simulink model "gm_soc_dvbs2_fpga"  (R2025b)
settings: Solver=VariableStepAuto  StartTime=0.0  StopTime=10.0  RelTol=1e-3
InitFcn:
  | soc_dvbs2_init;
undefined symbols (not defined in the file or in its folder): Add, coefficientsLog, coefficientsSqrt1, coefficientsSqrt2, dataBits, Deinterleaver, designMultirateFIR, noisePow, Shift, Short, soc_dvbs2_designFIRFilter, soc_dvbs2_txPacketBits, syncWord, txDataOut, txFiltCoeff, XData
libraries: simulink x304, hdlsllib x265, dspsigops x15, dsphdlfiltering2 x8, hdlmdlgenlib x6, dsphdlsigops2 x5, commseqgen3 x5, dsphdlmathfun2 x3, hwlogicconnlib x2, whdledac x2, commhdlcrc x2, whdlutilities x1
(part 27 of 36)

== system gm_soc_dvbs2_fpga/DVBS2/DVBS2 TxRx/DVB-S2 HDL Receiver/Synchronizer and PL Header Decoder/PL Header Recovery/PL Header Decoder/ML Decoder/Euclidean Distance Sum Up_instance55 ==
  note: For Each
  Ed0 : Inport  OutDataTypeStr=fixdt(1, 25, 15)  PortDimensions=1  SampleTime=2.5e-07
  Ed1 : Inport  Port=2  OutDataTypeStr=fixdt(1, 20, 13)  PortDimensions=1  SampleTime=2.5e-07
  reset : Inport  Port=3  OutDataTypeStr=boolean  PortDimensions=1  SampleTime=2.5e-07
  CWswitch : Inport  Port=4  OutDataTypeStr=fixdt(0, 1, 0)  PortDimensions=1  SampleTime=2.5e-07
  validIn : Inport  Port=5  OutDataTypeStr=boolean  PortDimensions=1  SampleTime=2.5e-07
  Add : Sum  OutDataTypeStr=fixdt(1, 25, 15)  AccumDataTypeStr=fixdt(1, 26, 15)  SampleTime=2.5e-07
  Delay{1..4} (4 alike) : Delay  DelayLength=double(1)  InitialCondition=0  SampleTime=2.5e-07
  Switch : Switch  Criteria=u2 ~= 0  Threshold="fi(0,0,1,0,\"hex\",\"0\")"  OutDataTypeStr=fixdt(1, 25, 15)  SampleTime=2.5e-07  SaturateOnIntegerOverflow=off  InputSameDT=off
  Unit Delay Enabled Resettable Synchronous : hdlsllib/Discrete/Unit Delay Enabled Resettable Synchronous  InitialCondition=double(0)  SampleTime=-1
  CwEdMetric : Outport  SampleTime=2.5e-07
  wires:
  Switch/1 -> Delay3/1
  validIn/1 -> Delay1/1
  Delay1/1 -> Unit Delay Enabled Resettable Synchronous/2
  Ed0/1 -> Switch/3
  reset/1 -> Delay2/1
  CWswitch/1 -> Switch/2
  Ed1/1 -> Switch/1
  Delay2/1 -> Unit Delay Enabled Resettable Synchronous/3
  Unit Delay Enabled Resettable Synchronous/1 -> Delay4/1, Add/1
  Add/1 -> Unit Delay Enabled Resettable Synchronous/1
  Delay3/1 -> Add/2
  Delay4/1 -> CwEdMetric/1

== system gm_soc_dvbs2_fpga/DVBS2/DVBS2 TxRx/DVB-S2 HDL Receiver/Synchronizer and PL Header Decoder/PL Header Recovery/PL Header Decoder/ML Decoder/Euclidean Distance Sum Up_instance56 ==
  note: For Each
  Ed0 : Inport  OutDataTypeStr=fixdt(1, 25, 15)  PortDimensions=1  SampleTime=2.5e-07
  Ed1 : Inport  Port=2  OutDataTypeStr=fixdt(1, 20, 13)  PortDimensions=1  SampleTime=2.5e-07
  reset : Inport  Port=3  OutDataTypeStr=boolean  PortDimensions=1  SampleTime=2.5e-07
  CWswitch : Inport  Port=4  OutDataTypeStr=fixdt(0, 1, 0)  PortDimensions=1  SampleTime=2.5e-07
  validIn : Inport  Port=5  OutDataTypeStr=boolean  PortDimensions=1  SampleTime=2.5e-07
  Add : Sum  OutDataTypeStr=fixdt(1, 25, 15)  AccumDataTypeStr=fixdt(1, 26, 15)  SampleTime=2.5e-07
  Delay{1..4} (4 alike) : Delay  DelayLength=double(1)  InitialCondition=0  SampleTime=2.5e-07
  Switch : Switch  Criteria=u2 ~= 0  Threshold="fi(0,0,1,0,\"hex\",\"0\")"  OutDataTypeStr=fixdt(1, 25, 15)  SampleTime=2.5e-07  SaturateOnIntegerOverflow=off  InputSameDT=off
  Unit Delay Enabled Resettable Synchronous : hdlsllib/Discrete/Unit Delay Enabled Resettable Synchronous  InitialCondition=double(0)  SampleTime=-1
  CwEdMetric : Outport  SampleTime=2.5e-07
  wires:
  validIn/1 -> Delay1/1
  Delay1/1 -> Unit Delay Enabled Resettable Synchronous/2
  Ed0/1 -> Switch/3
  reset/1 -> Delay2/1
  Delay2/1 -> Unit Delay Enabled Resettable Synchronous/3
  CWswitch/1 -> Switch/2
  Ed1/1 -> Switch/1
  Switch/1 -> Delay3/1
  Unit Delay Enabled Resettable Synchronous/1 -> Delay4/1, Add/1
  Delay3/1 -> Add/2
  Delay4/1 -> CwEdMetric/1
  Add/1 -> Unit Delay Enabled Resettable Synchronous/1

== system gm_soc_dvbs2_fpga/DVBS2/DVBS2 TxRx/DVB-S2 HDL Receiver/Synchronizer and PL Header Decoder/PL Header Recovery/PL Header Decoder/ML Decoder/Euclidean Distance Sum Up_instance57 ==
  note: For Each
  Ed0 : Inport  OutDataTypeStr=fixdt(1, 25, 15)  PortDimensions=1  SampleTime=2.5e-07
  Ed1 : Inport  Port=2  OutDataTypeStr=fixdt(1, 20, 13)  PortDimensions=1  SampleTime=2.5e-07
  reset : Inport  Port=3  OutDataTypeStr=boolean  PortDimensions=1  SampleTime=2.5e-07
  CWswitch : Inport  Port=4  OutDataTypeStr=fixdt(0, 1, 0)  PortDimensions=1  SampleTime=2.5e-07
  validIn : Inport  Port=5  OutDataTypeStr=boolean  PortDimensions=1  SampleTime=2.5e-07
  Add : Sum  OutDataTypeStr=fixdt(1, 25, 15)  AccumDataTypeStr=fixdt(1, 26, 15)  SampleTime=2.5e-07
  Delay{1..4} (4 alike) : Delay  DelayLength=double(1)  InitialCondition=0  SampleTime=2.5e-07
  Switch : Switch  Criteria=u2 ~= 0  Threshold="fi(0,0,1,0,\"hex\",\"0\")"  OutDataTypeStr=fixdt(1, 25, 15)  SampleTime=2.5e-07  SaturateOnIntegerOverflow=off  InputSameDT=off
  Unit Delay Enabled Resettable Synchronous : hdlsllib/Discrete/Unit Delay Enabled Resettable Synchronous  InitialCondition=double(0)  SampleTime=-1
  CwEdMetric : Outport  SampleTime=2.5e-07
  wires:
  Switch/1 -> Delay3/1
  validIn/1 -> Delay1/1
  Delay1/1 -> Unit Delay Enabled Resettable Synchronous/2
  Ed0/1 -> Switch/3
  reset/1 -> Delay2/1
  CWswitch/1 -> Switch/2
  Ed1/1 -> Switch/1
  Delay2/1 -> Unit Delay Enabled Resettable Synchronous/3
  Unit Delay Enabled Resettable Synchronous/1 -> Delay4/1, Add/1
  Add/1 -> Unit Delay Enabled Resettable Synchronous/1
  Delay3/1 -> Add/2
  Delay4/1 -> CwEdMetric/1

== system gm_soc_dvbs2_fpga/DVBS2/DVBS2 TxRx/DVB-S2 HDL Receiver/Synchronizer and PL Header Decoder/PL Header Recovery/PL Header Decoder/ML Decoder/Euclidean Distance Sum Up_instance58 ==
  note: For Each
  Ed0 : Inport  OutDataTypeStr=fixdt(1, 25, 15)  PortDimensions=1  SampleTime=2.5e-07
  Ed1 : Inport  Port=2  OutDataTypeStr=fixdt(1, 20, 13)  PortDimensions=1  SampleTime=2.5e-07
  reset : Inport  Port=3  OutDataTypeStr=boolean  PortDimensions=1  SampleTime=2.5e-07
  CWswitch : Inport  Port=4  OutDataTypeStr=fixdt(0, 1, 0)  PortDimensions=1  SampleTime=2.5e-07
  validIn : Inport  Port=5  OutDataTypeStr=boolean  PortDimensions=1  SampleTime=2.5e-07
  Add : Sum  OutDataTypeStr=fixdt(1, 25, 15)  AccumDataTypeStr=fixdt(1, 26, 15)  SampleTime=2.5e-07
  Delay{1..4} (4 alike) : Delay  DelayLength=double(1)  InitialCondition=0  SampleTime=2.5e-07
  Switch : Switch  Criteria=u2 ~= 0  Threshold="fi(0,0,1,0,\"hex\",\"0\")"  OutDataTypeStr=fixdt(1, 25, 15)  SampleTime=2.5e-07  SaturateOnIntegerOverflow=off  InputSameDT=off
  Unit Delay Enabled Resettable Synchronous : hdlsllib/Discrete/Unit Delay Enabled Resettable Synchronous  InitialCondition=double(0)  SampleTime=-1
  CwEdMetric : Outport  SampleTime=2.5e-07
  wires:
  Switch/1 -> Delay3/1
  validIn/1 -> Delay1/1
  Delay1/1 -> Unit Delay Enabled Resettable Synchronous/2
  Ed0/1 -> Switch/3
  reset/1 -> Delay2/1
  Delay2/1 -> Unit Delay Enabled Resettable Synchronous/3
  CWswitch/1 -> Switch/2
  Ed1/1 -> Switch/1
  Unit Delay Enabled Resettable Synchronous/1 -> Delay4/1, Add/1
  Delay3/1 -> Add/2
  Delay4/1 -> CwEdMetric/1
  Add/1 -> Unit Delay Enabled Resettable Synchronous/1

== system gm_soc_dvbs2_fpga/DVBS2/DVBS2 TxRx/DVB-S2 HDL Receiver/Synchronizer and PL Header Decoder/PL Header Recovery/PL Header Decoder/ML Decoder/Euclidean Distance Sum Up_instance59 ==
  note: For Each
  Ed0 : Inport  OutDataTypeStr=fixdt(1, 25, 15)  PortDimensions=1  SampleTime=2.5e-07
  Ed1 : Inport  Port=2  OutDataTypeStr=fixdt(1, 20, 13)  PortDimensions=1  SampleTime=2.5e-07
  reset : Inport  Port=3  OutDataTypeStr=boolean  PortDimensions=1  SampleTime=2.5e-07
  CWswitch : Inport  Port=4  OutDataTypeStr=fixdt(0, 1, 0)  PortDimensions=1  SampleTime=2.5e-07
  validIn : Inport  Port=5  OutDataTypeStr=boolean  PortDimensions=1  SampleTime=2.5e-07
  Add : Sum  OutDataTypeStr=fixdt(1, 25, 15)  AccumDataTypeStr=fixdt(1, 26, 15)  SampleTime=2.5e-07
  Delay{1..4} (4 alike) : Delay  DelayLength=double(1)  InitialCondition=0  SampleTime=2.5e-07
  Switch : Switch  Criteria=u2 ~= 0  Threshold="fi(0,0,1,0,\"hex\",\"0\")"  OutDataTypeStr=fixdt(1, 25, 15)  SampleTime=2.5e-07  SaturateOnIntegerOverflow=off  InputSameDT=off
  Unit Delay Enabled Resettable Synchronous : hdlsllib/Discrete/Unit Delay Enabled Resettable Synchronous  InitialCondition=double(0)  SampleTime=-1
  CwEdMetric : Outport  SampleTime=2.5e-07
  wires:
  Switch/1 -> Delay3/1
  validIn/1 -> Delay1/1
  Delay1/1 -> Unit Delay Enabled Resettable Synchronous/2
  Ed0/1 -> Switch/3
  reset/1 -> Delay2/1
  CWswitch/1 -> Switch/2
  Ed1/1 -> Switch/1
  Delay2/1 -> Unit Delay Enabled Resettable Synchronous/3
  Unit Delay Enabled Resettable Synchronous/1 -> Add/1, Delay4/1
  Add/1 -> Unit Delay Enabled Resettable Synchronous/1
  Delay3/1 -> Add/2
  Delay4/1 -> CwEdMetric/1

== system gm_soc_dvbs2_fpga/DVBS2/DVBS2 TxRx/DVB-S2 HDL Receiver/Synchronizer and PL Header Decoder/PL Header Recovery/PL Header Decoder/ML Decoder/Euclidean Distance Sum Up_instance6 ==
  note: For Each
  Ed0 : Inport  OutDataTypeStr=fixdt(1, 25, 15)  PortDimensions=1  SampleTime=2.5e-07
  Ed1 : Inport  Port=2  OutDataTypeStr=fixdt(1, 20, 13)  PortDimensions=1  SampleTime=2.5e-07
  reset : Inport  Port=3  OutDataTypeStr=boolean  PortDimensions=1  SampleTime=2.5e-07
  CWswitch : Inport  Port=4  OutDataTypeStr=fixdt(0, 1, 0)  PortDimensions=1  SampleTime=2.5e-07
  validIn : Inport  Port=5  OutDataTypeStr=boolean  PortDimensions=1  SampleTime=2.5e-07
  Add : Sum  OutDataTypeStr=fixdt(1, 25, 15)  AccumDataTypeStr=fixdt(1, 26, 15)  SampleTime=2.5e-07
  Delay{1..4} (4 alike) : Delay  DelayLength=double(1)  InitialCondition=0  SampleTime=2.5e-07
  Switch : Switch  Criteria=u2 ~= 0  Threshold="fi(0,0,1,0,\"hex\",\"0\")"  OutDataTypeStr=fixdt(1, 25, 15)  SampleTime=2.5e-07  SaturateOnIntegerOverflow=off  InputSameDT=off
  Unit Delay Enabled Resettable Synchronous : hdlsllib/Discrete/Unit Delay Enabled Resettable Synchronous  InitialCondition=double(0)  SampleTime=-1
  CwEdMetric : Outport  SampleTime=2.5e-07
  wires:
  Switch/1 -> Delay3/1
  validIn/1 -> Delay1/1
  Delay1/1 -> Unit Delay Enabled Resettable Synchronous/2
  Ed0/1 -> Switch/3
  reset/1 -> Delay2/1
  Delay2/1 -> Unit Delay Enabled Resettable Synchronous/3
  CWswitch/1 -> Switch/2
  Ed1/1 -> Switch/1
  Unit Delay Enabled Resettable Synchronous/1 -> Delay4/1, Add/1
  Add/1 -> Unit Delay Enabled Resettable Synchronous/1
  Delay3/1 -> Add/2
  Delay4/1 -> CwEdMetric/1

== system gm_soc_dvbs2_fpga/DVBS2/DVBS2 TxRx/DVB-S2 HDL Receiver/Synchronizer and PL Header Decoder/PL Header Recovery/PL Header Decoder/ML Decoder/Euclidean Distance Sum Up_instance60 ==
  note: For Each
  Ed0 : Inport  OutDataTypeStr=fixdt(1, 25, 15)  PortDimensions=1  SampleTime=2.5e-07
  Ed1 : Inport  Port=2  OutDataTypeStr=fixdt(1, 20, 13)  PortDimensions=1  SampleTime=2.5e-07
  reset : Inport  Port=3  OutDataTypeStr=boolean  PortDimensions=1  SampleTime=2.5e-07
  CWswitch : Inport  Port=4  OutDataTypeStr=fixdt(0, 1, 0)  PortDimensions=1  SampleTime=2.5e-07
  validIn : Inport  Port=5  OutDataTypeStr=boolean  PortDimensions=1  SampleTime=2.5e-07
  Add : Sum  OutDataTypeStr=fixdt(1, 25, 15)  AccumDataTypeStr=fixdt(1, 26, 15)  SampleTime=2.5e-07
  Delay{1..4} (4 alike) : Delay  DelayLength=double(1)  InitialCondition=0  SampleTime=2.5e-07
  Switch : Switch  Criteria=u2 ~= 0  Threshold="fi(0,0,1,0,\"hex\",\"0\")"  OutDataTypeStr=fixdt(1, 25, 15)  SampleTime=2.5e-07  SaturateOnIntegerOverflow=off  InputSameDT=off
  Unit Delay Enabled Resettable Synchronous : hdlsllib/Discrete/Unit Delay Enabled Resettable Synchronous  InitialCondition=double(0)  SampleTime=-1
  CwEdMetric : Outport  SampleTime=2.5e-07
  wires:
  Switch/1 -> Delay3/1
  validIn/1 -> Delay1/1
  Delay1/1 -> Unit Delay Enabled Resettable Synchronous/2
  Ed0/1 -> Switch/3
  reset/1 -> Delay2/1
  Delay2/1 -> Unit Delay Enabled Resettable Synchronous/3
  CWswitch/1 -> Switch/2
  Ed1/1 -> Switch/1
  Unit Delay Enabled Resettable Synchronous/1 -> Delay4/1, Add/1
  Delay3/1 -> Add/2
  Delay4/1 -> CwEdMetric/1
  Add/1 -> Unit Delay Enabled Resettable Synchronous/1

== system gm_soc_dvbs2_fpga/DVBS2/DVBS2 TxRx/DVB-S2 HDL Receiver/Synchronizer and PL Header Decoder/PL Header Recovery/PL Header Decoder/ML Decoder/Euclidean Distance Sum Up_instance61 ==
  note: For Each
  Ed0 : Inport  OutDataTypeStr=fixdt(1, 25, 15)  PortDimensions=1  SampleTime=2.5e-07
  Ed1 : Inport  Port=2  OutDataTypeStr=fixdt(1, 20, 13)  PortDimensions=1  SampleTime=2.5e-07
  reset : Inport  Port=3  OutDataTypeStr=boolean  PortDimensions=1  SampleTime=2.5e-07
  CWswitch : Inport  Port=4  OutDataTypeStr=fixdt(0, 1, 0)  PortDimensions=1  SampleTime=2.5e-07
  validIn : Inport  Port=5  OutDataTypeStr=boolean  PortDimensions=1  SampleTime=2.5e-07
  Add : Sum  OutDataTypeStr=fixdt(1, 25, 15)  AccumDataTypeStr=fixdt(1, 26, 15)  SampleTime=2.5e-07
  Delay{1..4} (4 alike) : Delay  DelayLength=double(1)  InitialCondition=0  SampleTime=2.5e-07
  Switch : Switch  Criteria=u2 ~= 0  Threshold="fi(0,0,1,0,\"hex\",\"0\")"  OutDataTypeStr=fixdt(1, 25, 15)  SampleTime=2.5e-07  SaturateOnIntegerOverflow=off  InputSameDT=off
  Unit Delay Enabled Resettable Synchronous : hdlsllib/Discrete/Unit Delay Enabled Resettable Synchronous  InitialCondition=double(0)  SampleTime=-1
  CwEdMetric : Outport  SampleTime=2.5e-07
  wires:
  Switch/1 -> Delay3/1
  validIn/1 -> Delay1/1
  Delay1/1 -> Unit Delay Enabled Resettable Synchronous/2
  Ed0/1 -> Switch/3
  reset/1 -> Delay2/1
  CWswitch/1 -> Switch/2
  Ed1/1 -> Switch/1
  Delay2/1 -> Unit Delay Enabled Resettable Synchronous/3
  Unit Delay Enabled Resettable Synchronous/1 -> Delay4/1, Add/1
  Add/1 -> Unit Delay Enabled Resettable Synchronous/1
  Delay3/1 -> Add/2
  Delay4/1 -> CwEdMetric/1

== system gm_soc_dvbs2_fpga/DVBS2/DVBS2 TxRx/DVB-S2 HDL Receiver/Synchronizer and PL Header Decoder/PL Header Recovery/PL Header Decoder/ML Decoder/Euclidean Distance Sum Up_instance62 ==
  note: For Each
  Ed0 : Inport  OutDataTypeStr=fixdt(1, 25, 15)  PortDimensions=1  SampleTime=2.5e-07
  Ed1 : Inport  Port=2  OutDataTypeStr=fixdt(1, 20, 13)  PortDimensions=1  SampleTime=2.5e-07
  reset : Inport  Port=3  OutDataTypeStr=boolean  PortDimensions=1  SampleTime=2.5e-07
  CWswitch : Inport  Port=4  OutDataTypeStr=fixdt(0, 1, 0)  PortDimensions=1  SampleTime=2.5e-07
  validIn : Inport  Port=5  OutDataTypeStr=boolean  PortDimensions=1  SampleTime=2.5e-07
  Add : Sum  OutDataTypeStr=fixdt(1, 25, 15)  AccumDataTypeStr=fixdt(1, 26, 15)  SampleTime=2.5e-07
  Delay{1..4} (4 alike) : Delay  DelayLength=double(1)  InitialCondition=0  SampleTime=2.5e-07
  Switch : Switch  Criteria=u2 ~= 0  Threshold="fi(0,0,1,0,\"hex\",\"0\")"  OutDataTypeStr=fixdt(1, 25, 15)  SampleTime=2.5e-07  SaturateOnIntegerOverflow=off  InputSameDT=off
  Unit Delay Enabled Resettable Synchronous : hdlsllib/Discrete/Unit Delay Enabled Resettable Synchronous  InitialCondition=double(0)  SampleTime=-1
  CwEdMetric : Outport  SampleTime=2.5e-07
  wires:
  Switch/1 -> Delay3/1
  validIn/1 -> Delay1/1
  Delay1/1 -> Unit Delay Enabled Resettable Synchronous/2
  Ed0/1 -> Switch/3
  reset/1 -> Delay2/1
  Delay2/1 -> Unit Delay Enabled Resettable Synchronous/3
  CWswitch/1 -> Switch/2
  Ed1/1 -> Switch/1
  Unit Delay Enabled Resettable Synchronous/1 -> Add/1, Delay4/1
  Add/1 -> Unit Delay Enabled Resettable Synchronous/1
  Delay3/1 -> Add/2
  Delay4/1 -> CwEdMetric/1

== system gm_soc_dvbs2_fpga/DVBS2/DVBS2 TxRx/DVB-S2 HDL Receiver/Synchronizer and PL Header Decoder/PL Header Recovery/PL Header Decoder/ML Decoder/Euclidean Distance Sum Up_instance63 ==
  note: For Each
  Ed0 : Inport  OutDataTypeStr=fixdt(1, 25, 15)  PortDimensions=1  SampleTime=2.5e-07
  Ed1 : Inport  Port=2  OutDataTypeStr=fixdt(1, 20, 13)  PortDimensions=1  SampleTime=2.5e-07
  reset : Inport  Port=3  OutDataTypeStr=boolean  PortDimensions=1  SampleTime=2.5e-07
  CWswitch : Inport  Port=4  OutDataTypeStr=fixdt(0, 1, 0)  PortDimensions=1  SampleTime=2.5e-07
  validIn : Inport  Port=5  OutDataTypeStr=boolean  PortDimensions=1  SampleTime=2.5e-07
  Add : Sum  OutDataTypeStr=fixdt(1, 25, 15)  AccumDataTypeStr=fixdt(1, 26, 15)  SampleTime=2.5e-07
  Delay{1..4} (4 alike) : Delay  DelayLength=double(1)  InitialCondition=0  SampleTime=2.5e-07
  Switch : Switch  Criteria=u2 ~= 0  Threshold="fi(0,0,1,0,\"hex\",\"0\")"  OutDataTypeStr=fixdt(1, 25, 15)  SampleTime=2.5e-07  SaturateOnIntegerOverflow=off  InputSameDT=off
  Unit Delay Enabled Resettable Synchronous : hdlsllib/Discrete/Unit Delay Enabled Resettable Synchronous  InitialCondition=double(0)  SampleTime=-1
  CwEdMetric : Outport  SampleTime=2.5e-07
  wires:
  Switch/1 -> Delay3/1
  validIn/1 -> Delay1/1
  Delay1/1 -> Unit Delay Enabled Resettable Synchronous/2
  Ed0/1 -> Switch/3
  reset/1 -> Delay2/1
  CWswitch/1 -> Switch/2
  Ed1/1 -> Switch/1
  Delay2/1 -> Unit Delay Enabled Resettable Synchronous/3
  Unit Delay Enabled Resettable Synchronous/1 -> Add/1, Delay4/1
  Add/1 -> Unit Delay Enabled Resettable Synchronous/1
  Delay3/1 -> Add/2
  Delay4/1 -> CwEdMetric/1

== system gm_soc_dvbs2_fpga/DVBS2/DVBS2 TxRx/DVB-S2 HDL Receiver/Synchronizer and PL Header Decoder/PL Header Recovery/PL Header Decoder/ML Decoder/Euclidean Distance Sum Up_instance64 ==
  note: For Each
  Ed0 : Inport  OutDataTypeStr=fixdt(1, 25, 15)  PortDimensions=1  SampleTime=2.5e-07
  Ed1 : Inport  Port=2  OutDataTypeStr=fixdt(1, 20, 13)  PortDimensions=1  SampleTime=2.5e-07
  reset : Inport  Port=3  OutDataTypeStr=boolean  PortDimensions=1  SampleTime=2.5e-07
  CWswitch : Inport  Port=4  OutDataTypeStr=fixdt(0, 1, 0)  PortDimensions=1  SampleTime=2.5e-07
  validIn : Inport  Port=5  OutDataTypeStr=boolean  PortDimensions=1  SampleTime=2.5e-07
  Add : Sum  OutDataTypeStr=fixdt(1, 25, 15)  AccumDataTypeStr=fixdt(1, 26, 15)  SampleTime=2.5e-07
  Delay{1..4} (4 alike) : Delay  DelayLength=double(1)  InitialCondition=0  SampleTime=2.5e-07
  Switch : Switch  Criteria=u2 ~= 0  Threshold="fi(0,0,1,0,\"hex\",\"0\")"  OutDataTypeStr=fixdt(1, 25, 15)  SampleTime=2.5e-07  SaturateOnIntegerOverflow=off  InputSameDT=off
  Unit Delay Enabled Resettable Synchronous : hdlsllib/Discrete/Unit Delay Enabled Resettable Synchronous  InitialCondition=double(0)  SampleTime=-1
  CwEdMetric : Outport  SampleTime=2.5e-07
  wires:
  Switch/1 -> Delay3/1
  validIn/1 -> Delay1/1
  Delay1/1 -> Unit Delay Enabled Resettable Synchronous/2
  Ed0/1 -> Switch/3
  reset/1 -> Delay2/1
  Delay2/1 -> Unit Delay Enabled Resettable Synchronous/3
  CWswitch/1 -> Switch/2
  Ed1/1 -> Switch/1
  Unit Delay Enabled Resettable Synchronous/1 -> Delay4/1, Add/1
  Add/1 -> Unit Delay Enabled Resettable Synchronous/1
  Delay3/1 -> Add/2
  Delay4/1 -> CwEdMetric/1

== system gm_soc_dvbs2_fpga/DVBS2/DVBS2 TxRx/DVB-S2 HDL Receiver/Synchronizer and PL Header Decoder/PL Header Recovery/PL Header Decoder/ML Decoder/Euclidean Distance Sum Up_instance7 ==
  note: For Each
  Ed0 : Inport  OutDataTypeStr=fixdt(1, 25, 15)  PortDimensions=1  SampleTime=2.5e-07
  Ed1 : Inport  Port=2  OutDataTypeStr=fixdt(1, 20, 13)  PortDimensions=1  SampleTime=2.5e-07
  reset : Inport  Port=3  OutDataTypeStr=boolean  PortDimensions=1  SampleTime=2.5e-07
  CWswitch : Inport  Port=4  OutDataTypeStr=fixdt(0, 1, 0)  PortDimensions=1  SampleTime=2.5e-07
  validIn : Inport  Port=5  OutDataTypeStr=boolean  PortDimensions=1  SampleTime=2.5e-07
  Add : Sum  OutDataTypeStr=fixdt(1, 25, 15)  AccumDataTypeStr=fixdt(1, 26, 15)  SampleTime=2.5e-07
  Delay{1..4} (4 alike) : Delay  DelayLength=double(1)  InitialCondition=0  SampleTime=2.5e-07
  Switch : Switch  Criteria=u2 ~= 0  Threshold="fi(0,0,1,0,\"hex\",\"0\")"  OutDataTypeStr=fixdt(1, 25, 15)  SampleTime=2.5e-07  SaturateOnIntegerOverflow=off  InputSameDT=off
  Unit Delay Enabled Resettable Synchronous : hdlsllib/Discrete/Unit Delay Enabled Resettable Synchronous  InitialCondition=double(0)  SampleTime=-1
  CwEdMetric : Outport  SampleTime=2.5e-07
  wires:
  Ed0/1 -> Switch/3
  reset/1 -> Delay2/1
  validIn/1 -> Delay1/1
  CWswitch/1 -> Switch/2
  Ed1/1 -> Switch/1
  Switch/1 -> Delay3/1
  Delay1/1 -> Unit Delay Enabled Resettable Synchronous/2
  Delay2/1 -> Unit Delay Enabled Resettable Synchronous/3
  Unit Delay Enabled Resettable Synchronous/1 -> Delay4/1, Add/1
  Add/1 -> Unit Delay Enabled Resettable Synchronous/1
  Delay3/1 -> Add/2
  Delay4/1 -> CwEdMetric/1

== system gm_soc_dvbs2_fpga/DVBS2/DVBS2 TxRx/DVB-S2 HDL Receiver/Synchronizer and PL Header Decoder/PL Header Recovery/PL Header Decoder/ML Decoder/Euclidean Distance Sum Up_instance8 ==
  note: For Each
  Ed0 : Inport  OutDataTypeStr=fixdt(1, 25, 15)  PortDimensions=1  SampleTime=2.5e-07
  Ed1 : Inport  Port=2  OutDataTypeStr=fixdt(1, 20, 13)  PortDimensions=1  SampleTime=2.5e-07
  reset : Inport  Port=3  OutDataTypeStr=boolean  PortDimensions=1  SampleTime=2.5e-07
  CWswitch : Inport  Port=4  OutDataTypeStr=fixdt(0, 1, 0)  PortDimensions=1  SampleTime=2.5e-07
  validIn : Inport  Port=5  OutDataTypeStr=boolean  PortDimensions=1  SampleTime=2.5e-07
  Add : Sum  OutDataTypeStr=fixdt(1, 25, 15)  AccumDataTypeStr=fixdt(1, 26, 15)  SampleTime=2.5e-07
  Delay{1..4} (4 alike) : Delay  DelayLength=double(1)  InitialCondition=0  SampleTime=2.5e-07
  Switch : Switch  Criteria=u2 ~= 0  Threshold="fi(0,0,1,0,\"hex\",\"0\")"  OutDataTypeStr=fixdt(1, 25, 15)  SampleTime=2.5e-07  SaturateOnIntegerOverflow=off  InputSameDT=off
  Unit Delay Enabled Resettable Synchronous : hdlsllib/Discrete/Unit Delay Enabled Resettable Synchronous  InitialCondition=double(0)  SampleTime=-1
  CwEdMetric : Outport  SampleTime=2.5e-07
  wires:
  Switch/1 -> Delay3/1
  validIn/1 -> Delay1/1
  Delay1/1 -> Unit Delay Enabled Resettable Synchronous/2
  Ed0/1 -> Switch/3
  reset/1 -> Delay2/1
  Delay2/1 -> Unit Delay Enabled Resettable Synchronous/3
  CWswitch/1 -> Switch/2
  Ed1/1 -> Switch/1
  Unit Delay Enabled Resettable Synchronous/1 -> Delay4/1, Add/1
  Add/1 -> Unit Delay Enabled Resettable Synchronous/1
  Delay3/1 -> Add/2
  Delay4/1 -> CwEdMetric/1

== system gm_soc_dvbs2_fpga/DVBS2/DVBS2 TxRx/DVB-S2 HDL Receiver/Synchronizer and PL Header Decoder/PL Header Recovery/PL Header Decoder/ML Decoder/Euclidean Distance Sum Up_instance9 ==
  note: For Each
  Ed0 : Inport  OutDataTypeStr=fixdt(1, 25, 15)  PortDimensions=1  SampleTime=2.5e-07
  Ed1 : Inport  Port=2  OutDataTypeStr=fixdt(1, 20, 13)  PortDimensions=1  SampleTime=2.5e-07
  reset : Inport  Port=3  OutDataTypeStr=boolean  PortDimensions=1  SampleTime=2.5e-07
  CWswitch : Inport  Port=4  OutDataTypeStr=fixdt(0, 1, 0)  PortDimensions=1  SampleTime=2.5e-07
  validIn : Inport  Port=5  OutDataTypeStr=boolean  PortDimensions=1  SampleTime=2.5e-07
  Add : Sum  OutDataTypeStr=fixdt(1, 25, 15)  AccumDataTypeStr=fixdt(1, 26, 15)  SampleTime=2.5e-07
  Delay{1..4} (4 alike) : Delay  DelayLength=double(1)  InitialCondition=0  SampleTime=2.5e-07
  Switch : Switch  Criteria=u2 ~= 0  Threshold="fi(0,0,1,0,\"hex\",\"0\")"  OutDataTypeStr=fixdt(1, 25, 15)  SampleTime=2.5e-07  SaturateOnIntegerOverflow=off  InputSameDT=off
  Unit Delay Enabled Resettable Synchronous : hdlsllib/Discrete/Unit Delay Enabled Resettable Synchronous  InitialCondition=double(0)  SampleTime=-1
  CwEdMetric : Outport  SampleTime=2.5e-07
  wires:
  Ed0/1 -> Switch/3
  reset/1 -> Delay2/1
  validIn/1 -> Delay1/1
  CWswitch/1 -> Switch/2
  Ed1/1 -> Switch/1
  Switch/1 -> Delay3/1
  Delay1/1 -> Unit Delay Enabled Resettable Synchronous/2
  Delay2/1 -> Unit Delay Enabled Resettable Synchronous/3
  Unit Delay Enabled Resettable Synchronous/1 -> Delay4/1, Add/1
  Add/1 -> Unit Delay Enabled Resettable Synchronous/1
  Delay3/1 -> Add/2
  Delay4/1 -> CwEdMetric/1
